simulink model "test_HEx2_mod"  (R2016a)
settings: Solver=ode15s  StartTime=0.0  StopTime=1e5  MaxStep=1e2  RelTol=1e-3
libraries: simCryogenics_lib x18, nesl_utility x18
settings Model: Creator=SK248285  LastModifiedBy=SK248285
settings DataIOCC: LimitDataPoints=on  SaveFormat=Array  SaveState=on
settings HardwareCC: ProdBitPerPointer=32  ProdLargestAtomicFloat=None  ProdIntDivRoundTo=Undefined  ProdEndianess=Unspecified  ProdWordSize=32  ProdHWDeviceType=32-bit Generic
settings ModelReferenceCC: PropagateSignalLabelsOutOfModel=off
settings ConfigComp: CovModelRefEnable=Off
settings SimscapeCC: SimscapeLogType=all  SimscapeLogLimitData=off

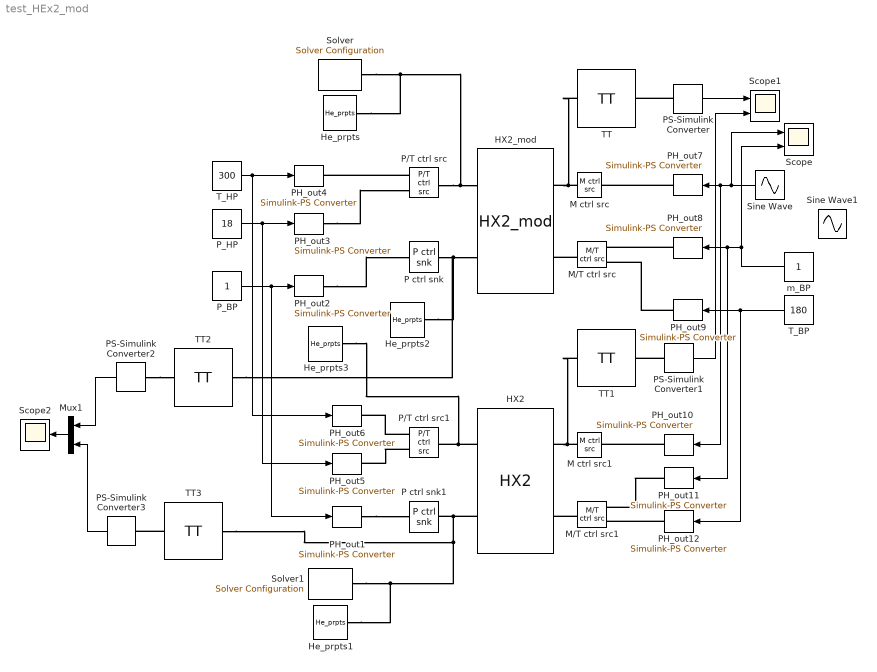
== system test_HEx2_mod ==
  HX2 : simCryogenics_lib/Elements/HX2  N=10  Vh=0.5 m^3  Vc=0.5 m^3  M=1000 kg  Kh=0 s*bar/kg  Kc=0 s*bar/kg  h=480000*2/8 J/s/K  Th0=300 K  Ph0=18 bar  Mh0=1 kg/s  Tc0=180 K  Pc0=1 bar  Mc0=1 kg/s
  HX2_mod : simCryogenics_lib/Elements/HX2_mod  N=10  Vh=0.5 m^3  Vc=0.5 m^3  M=1000 kg  Kh=0 s*bar/kg  Kc=0 s*bar/kg  Th0=300 K  Ph0=18 bar  Mh0=1 kg/s  Tc0=180 K  Pc0=1 bar  Mc0=1 kg/s  hhn=480000*2/8 J/s/K  hcn=480000*2/8 J/s/K  Mhn=1 kg/s  Mcn=1 kg/s  Thn=300 K  Tcn=180 K  Phn=18 bar  Pcn=1 bar  ex_mode=1
  He_prpts{,1..3} (4 alike) : simCryogenics_lib/Utilities/He_prpts  P_min=0.01 bar  P_max=20 bar  T_min=1.8 K  T_max=400 K  N=100  Mol=4.0026 * 10 ^ (- 3) kg/mol
  M ctrl src : simCryogenics_lib/Sources_Sinks/M ctrl src
  M ctrl src1 : simCryogenics_lib/Sources_Sinks/M ctrl src
  M/T ctrl src : simCryogenics_lib/Sources_Sinks/M//T ctrl src
  M/T ctrl src1 : simCryogenics_lib/Sources_Sinks/M//T ctrl src
  Mux1 : Mux  Inputs=2
  P ctrl snk : simCryogenics_lib/Sources_Sinks/P ctrl snk
  P ctrl snk1 : simCryogenics_lib/Sources_Sinks/P ctrl snk
  P/T ctrl src : simCryogenics_lib/Sources_Sinks/P//T ctrl src
  P/T ctrl src1 : simCryogenics_lib/Sources_Sinks/P//T ctrl src
  PH_out{1..3,5} (4 alike) : nesl_utility/Simulink-PS Converter  PhysicalDomain=network_engine_domain  SubClassName=ps_input  LeftPortType=input  RightPortType=output  PseudoPeriodic=off  Frequencies=[]  NoiseDistribution=none  NoiseParameters=[]  Unit=bar  AffineConversion=off  InputFiltering=off  SimscapeFilterOrder=1  InputFilterTimeConstant=0.001  UdotUserProvided=1
  PH_out{7..8,10..11} (4 alike) : nesl_utility/Simulink-PS Converter  PhysicalDomain=network_engine_domain  SubClassName=ps_input  LeftPortType=input  RightPortType=output  PseudoPeriodic=off  Frequencies=[]  NoiseDistribution=none  NoiseParameters=[]  Unit=kg/s  AffineConversion=off  InputFiltering=off  SimscapeFilterOrder=1  InputFilterTimeConstant=0.001  UdotUserProvided=1
  PH_out{4,6,9,12} (4 alike) : nesl_utility/Simulink-PS Converter  PhysicalDomain=network_engine_domain  SubClassName=ps_input  LeftPortType=input  RightPortType=output  PseudoPeriodic=off  Frequencies=[]  NoiseDistribution=none  NoiseParameters=[]  Unit=K  AffineConversion=off  InputFiltering=off  SimscapeFilterOrder=1  InputFilterTimeConstant=0.001  UdotUserProvided=1
  PS-Simulink Converter{,1..3} (4 alike) : nesl_utility/PS-Simulink Converter  PhysicalDomain=network_engine_domain  SubClassName=ps_output  LeftPortType=input  RightPortType=output  PseudoPeriodic=off  Frequencies=[]  Unit=1  AffineConversion=off
  P_BP : Constant
  P_HP : Constant  Value=18
  Scope : Scope  NumInputPorts=2
  Scope1 : Scope  NumInputPorts=2
  Scope2 : Scope
  Sine Wave : Sin  Bias=1  Frequency=1/1e5*2*pi  SampleTime=0
  Sine Wave1 : Sin  Bias=1  Frequency=1/1e5*2*pi  Phase=2*pi/16  SampleTime=0
  Solver : nesl_utility/Solver Configuration  PhysicalDomain=network_engine_domain  SubClassName=solver  LeftPortType=input  RightPortType=generic  Accelerate=off  Tones=[]  Harmonics=[]  SimulateNoise=off  Profile=off  UseLocalSampling=off  EnableSwitchedLinearOptims=on  FrequencyDomain=off  UseCCode=off  RelTol=0.001  AbsTol=1e-06  MinStep=1e-09  ToWorkspace=off  RevertToSquareIcSolve=off  NumHomotopyIterations=100  PhasorMode=off  PhasorModeNumHarmonics=1  OverrideAbsTol=off  DoDC=off  ResidualTolerance=1e9  UseLocalSolver=off  LocalSolverChoice=NE_BACKWARD_EULER_ADVANCER  LocalSolverSampleTime=5  DoFixedCost=off  MaxNonlinIter=3  MaxModeIter=2  LinearAlgebra=Sparse  DelaysMemoryBudget=1024  AutomaticFiltering=on  FilteringTimeConstant=0.001
  Solver1 : nesl_utility/Solver Configuration  PhysicalDomain=network_engine_domain  SubClassName=solver  LeftPortType=input  RightPortType=generic  Accelerate=off  Tones=[]  Harmonics=[]  SimulateNoise=off  Profile=off  UseLocalSampling=off  EnableSwitchedLinearOptims=on  FrequencyDomain=off  UseCCode=off  RelTol=0.001  AbsTol=1e-06  MinStep=1e-09  ToWorkspace=off  RevertToSquareIcSolve=off  NumHomotopyIterations=100  PhasorMode=off  PhasorModeNumHarmonics=1  OverrideAbsTol=off  DoDC=off  ResidualTolerance=1e-02  UseLocalSolver=off  LocalSolverChoice=NE_BACKWARD_EULER_ADVANCER  LocalSolverSampleTime=5  DoFixedCost=off  MaxNonlinIter=3  MaxModeIter=2  LinearAlgebra=Sparse  DelaysMemoryBudget=1024  AutomaticFiltering=on  FilteringTimeConstant=0.001
  TT{,1..3} (4 alike) : simCryogenics_lib/Sensors/TT
  T_BP : Constant  Value=180
  T_HP : Constant  Value=300
  m_BP : Constant
  wires:
  T_HP/1 -> PH_out4/1, PH_out6/1
  P_BP/1 -> PH_out1/1, PH_out2/1
  P_HP/1 -> PH_out5/1, PH_out3/1
  T_BP/1 -> PH_out12/1, PH_out9/1
  PS-Simulink Converter/1 -> Scope1/1
  PS-Simulink Converter1/1 -> Scope1/2
  PS-Simulink Converter2/1 -> Mux1/1
  Mux1/1 -> Scope2/1
  PS-Simulink Converter3/1 -> Mux1/2
  Sine Wave/1 -> Scope/1, PH_out10/1, PH_out7/1
  m_BP/1 -> Scope/2, PH_out11/1, PH_out8/1
  connections:
  P ctrl snk/RConn1 -- TT2/LConn1 -- He_prpts2/RConn1 -- HX2_mod/LConn1
  PH_out3/RConn1 -- P/T ctrl src/LConn1
  PH_out2/RConn1 -- P ctrl snk/LConn1
  P/T ctrl src/LConn2 -- PH_out4/RConn1
  M ctrl src/RConn1 -- TT/LConn1 -- HX2_mod/RConn2
  Solver/RConn1 -- HX2_mod/LConn2 -- P/T ctrl src/RConn1 -- He_prpts/RConn1
  M/T ctrl src/RConn1 -- HX2_mod/RConn1
  HX2/LConn2 -- He_prpts3/RConn1 -- P/T ctrl src1/RConn1
  Solver1/RConn1 -- TT3/LConn1 -- P ctrl snk1/RConn1 -- HX2/LConn1 -- He_prpts1/RConn1
  M/T ctrl src1/RConn1 -- HX2/RConn1
  M ctrl src1/RConn1 -- TT1/LConn1 -- HX2/RConn2
  PH_out7/RConn1 -- M ctrl src/LConn1
  PH_out8/RConn1 -- M/T ctrl src/LConn1
  PH_out9/RConn1 -- M/T ctrl src/LConn2
  P/T ctrl src1/LConn2 -- PH_out6/RConn1
  P/T ctrl src1/LConn1 -- PH_out5/RConn1
  PH_out1/RConn1 -- P ctrl snk1/LConn1
  PH_out10/RConn1 -- M ctrl src1/LConn1
  PH_out11/RConn1 -- M/T ctrl src1/LConn1
  PH_out12/RConn1 -- M/T ctrl src1/LConn2
  PS-Simulink Converter/LConn1 -- TT/RConn1
  PS-Simulink Converter1/LConn1 -- TT1/RConn1
  PS-Simulink Converter2/LConn1 -- TT2/RConn1
  TT3/RConn1 -- PS-Simulink Converter3/LConn1
